simulink model "ofdm"  (R2017b)
settings: Solver=FixedStepDiscrete  StartTime=0.0  StopTime=0.1  RelTol=1e-3
PreLoadFcn:
  | B=18e6;
  | driverChannels = 32;
  | dataChannels = 4096-driverChannels;
  | totalChannels = 4*4096;
  | tau = 100e-9;
  | SNR=30;
  | M=128;
  | Ts = (driverChannels+dataChannels)/B;
InitFcn:
  | B=18e6;
  | driverChannels = 32;
  | dataChannels = 4096-driverChannels;
  | totalChannels = 4096;
  | tau = 100e-9;
  | SNR=15;
  | M=4;
  | Ts = (driverChannels+dataChannels)/B;
undefined symbols (not defined in the file or in its folder): Channels, doppler
libraries: commchan3 x2, dspxfrm3 x2, commdigbbndam3 x2, commrandsrc3 x1, simulink x1, commsink2 x1, dspmathops x1
settings Model: SimulationMode=accelerator  Creator=nschrader  LastModifiedBy=nick
settings SolverCC: AutoInsertRateTranBlk=on
settings DataIOCC: LimitDataPoints=on  SaveOutput=off  SignalLogging=off  SaveTime=off
settings OptimizationCC: LifeSpan=inf
settings DebuggingCC: AlgebraicLoopMsg=error  SingleTaskRateTransMsg=error  AllowSymbolicDim=off  SFUnexpectedBacktrackingDiag=warning  SFNoUnconditionalDefaultTransitionDiag=warning  SFExecutionAtInitializationDiag=none
settings HardwareCC: ProdBitPerLong=64  ProdHWDeviceType=Intel->x86-64 (Linux 64)
settings CodeAppCC: StateflowObjectComments=on
settings GRTTargetCC: TargetLangStandard=C89/C90 (ANSI)  GeneratePreprocessorConditionals=Disable all

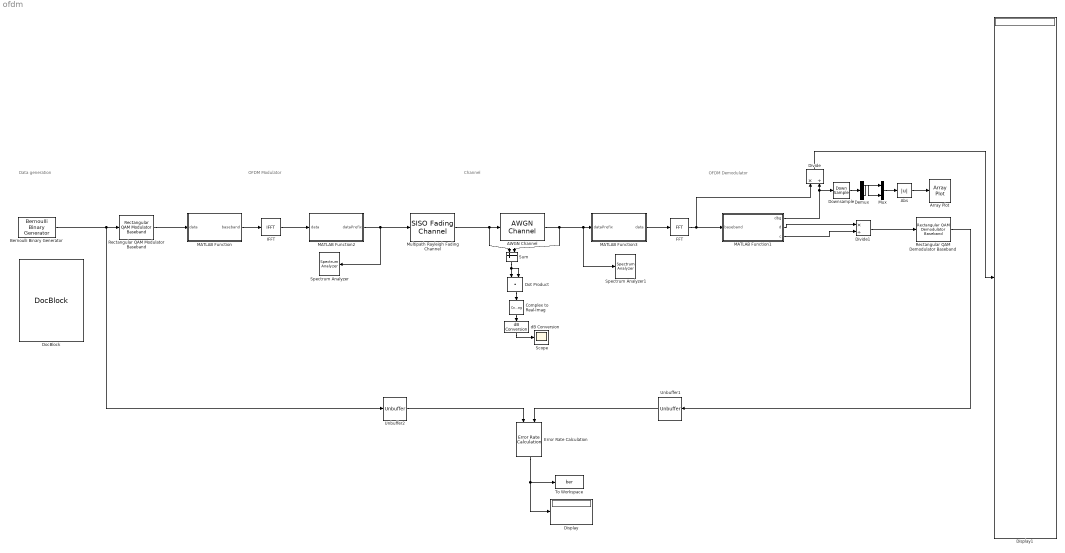
== system ofdm ==
  note: Data generation
  note: OFDM Modulator
  note: Channel
  note: OFDM Demodulator
  AWGN Channel : commchan3/AWGN Channel  InputProcessing=Columns as channels (frame based)  seed=67  noiseMode="Signal to noise ratio  (SNR)"  EbNodB=10  EsNodB=10  SNRdB=SNR  bitsPerSym=1  Ps=(driverChannels+dataChannels)/((totalChannels)^2)  Tsym=1  variance=1
  Abs : Abs
  Array Plot : ArrayPlot
  Bernoulli Binary Generator : commrandsrc3/Bernoulli Binary Generator  ProbabilityOfZero=0.5  SeedSource=Auto  Seed=0  SampleTime=Ts/dataChannels/log2(M)  SamplesPerFrame=dataChannels*log2(M)  OutputDataType=double  SimulateUsing=Code generation
  Complex to Real-Imag : ComplexToRealImag  Output=Real
  Demux : Demux  Outputs=2
  Display : Display
  Display1 : Display
  Divide : Product  Inputs=*/
  Divide1 : Product  Inputs=*/
  DocBlock : simulink/Model-Wide Utilities/DocBlock  DocumentType=Text  mask(DocBlock){}
      content=|
      | Type your documentation here
      mask Display:
      | B = evalin('base', 'B');
      | fprintf(['B = ',num2str(B*1e-6),' MHz\n\n\n\n\n\n\n\n\n\n\n\n\n\n\n\n']);
      | 
      | dataChannels = evalin('base', 'dataChannels');
      | fprintf(['dataChannels = ',num2str(dataChannels), '\n\n\n\n\n\n\n\n\n\n\n\n\n\n']);
      | 
      | totalChannels = evalin('base', 'totalChannels');
      | fprintf(['totalChannels = ',num2str(totalChannels), '\n\n\n\n\n\n\n\n\n\n\n\n']);
      | 
      | driverChannels = evalin('base', 'driverChannels');
      | fprintf(['driverChannels = ',num2str(driverChannels), '\n\n\n\n\n\n\n\n\n\n']);
      | 
      | SNR = evalin('base', 'SNR');
      | fprintf(['SNR = ',num2str(SNR), '\n\n\n\n\n\n\n\n']);
      | 
      | M = evalin('base', 'M');
      | fprintf(['M = ',num2str(M), '\n\n\n\n\n\n']);
      | 
      | Ts = evalin('base', 'Ts');
      | fprintf(['=> Ts = ',num2str(Ts*1e6), ' µs\n\n\n\n']);
      | 
      | rate = log2(M)*dataChannels/Ts/1e6;
      | fprintf(['=> dataRate = ',num2str(rate), ' Mbit/s\n\n']);
      | 
      | capacity = 20*log2(1+10^(SNR/10));
      | fprintf(['=> Efficientcy = ',num2str(100*rate/capacity), ' %%']);
  Dot Product : DotProduct  InputSameDT=on  OutDataTypeStr=Inherit: Inherit via internal rule
  Downsample : DownSample  N=32
  Error Rate Calculation : commsink2/Error Rate Calculation  N=0  st_delay=0  cp_mode=Entire frame  subframe=[]  PMode=Port  WsName=ErrorVec  RsMode2=off  stop=off  numErr=100  maxBits=1e6
  FFT : dspxfrm3/FFT  FFTImplementation=Auto  CompMethod=Table lookup  TableOpt=NEW  TableOptActive=Speed  BitRevOrder=off  Normalize=off  InheritFFTLength=on  FFTLength=Channels  WrapInput=off  roundingMode=Floor  overflowMode=off  firstCoeffDataTypeStr=Inherit: Same word length as input  firstCoeffLastDataTypeStr=Inherit: Same word length as input  outputMin=[]  outputMax=[]
  IFFT : dspxfrm3/IFFT  FFTImplementation=Auto  CompMethod=Table lookup  TableOpt=NEW  TableOptActive=Speed  BitRevOrder=off  cs_in=off  Normalize=on  InheritFFTLength=on  FFTLength=Channels*4  WrapInput=on  mode=Complex  outSamplingMode=Sample based  roundingMode=Floor  overflowMode=off  firstCoeffDataTypeStr=Inherit: Same word length as input  firstCoeffLastDataTypeStr=Inherit: Same word length as input  outputMin=[]  outputMax=[]
      settings: SourceProductName=DSP System Toolbox
  MATLAB Function : MATLAB Function  TreatAsAtomicUnit=on
  MATLAB Function1 : MATLAB Function  TreatAsAtomicUnit=on
  MATLAB Function2 : MATLAB Function  TreatAsAtomicUnit=on
  MATLAB Function3 : MATLAB Function  TreatAsAtomicUnit=on
  Multipath Rayleigh Fading Channel : commchan3/SISO Fading Channel  PathDelays=[0 0.5e-7 1e-7]  AveragePathGains=[0 -3 -6]  NormalizePathGains=on  FadingDistribution=Rayleigh  KFactor=3  DirectPathDopplerShift=0  DirectPathInitialPhase=0  MaximumDopplerShift=40  DopplerSpectrum=doppler('Jakes')  RandomStream=mt19937ar with seed  RandomNumGenerator=shr3cong  Seed=73  PathGainsOutputPort=off  ChannelFilterDelayOutputPort=off  SimulateUsing=Interpreted execution  Visualization=Off  PathsForDopplerDisplay=1  SamplesToDisplay=25%
      settings: SourceProductName=Communications System Toolbox
  Mux : Mux  Inputs=2
  Rectangular QAM Demodulator Baseband : commdigbbndam3/Rectangular QAM Demodulator Baseband  M=M  OutType=Bit  DecType=Hard decision  VarSource=Dialog  Variance=1  Dec=Gray  Mapping=[0:15]  PowType=Average Power  MinDist=2  AvgPow=1  PeakPow=1  Ph=0  outDtype1=Inherit via internal rule  outDtype2=Inherit via internal rule  derotateFactorWordLen=16  derotateFactorDataTypeStr=Inherit: Same word length as input  derotateFactorLastDataTypeStr=Inherit: Same word length as input  denormFactorWordLen=16  denormFactorDataTypeStr=Inherit: Same word length as input  denormFactorLastDataTypeStr=Inherit: Same word length as input  prodOutWordLen=32  prodOutOverflowMode=Wrap  prodOutRoundingMode=Floor  prodOutOvFlMode=off  prodOutOvFlModeLastStrValue=off  sumWordLen=32
  Rectangular QAM Modulator Baseband : commdigbbndam3/Rectangular QAM Modulator Baseband  M=M  InType=Bit  Enc=Gray  Mapping=[0:15]  PowType=Average Power  MinDist=2  AvgPow=1  PeakPow=1  Ph=0  outDtype=double  outWordLen=16  outUDDataType=sfix(16)  outFracLenMode=Best precision  outFracLen=15  outDataTypeStr=double  outLastDataTypeStr=double
  Scope : Scope
  Spectrum Analyzer : SpectrumAnalyzer
  Spectrum Analyzer1 : SpectrumAnalyzer
  Sum : Sum  Inputs=+-
  To Workspace : ToWorkspace  VariableName=ber  SaveFormat=Timeseries  SampleTime=-1
  Unbuffer1 : Unbuffer
  Unbuffer2 : Unbuffer
  dB Conversion : dspmathops/dB Conversion  dBtype=dB  intype=Power  R=1  fuzz=off
      settings: SourceProductName=DSP System Toolbox
  wires:
  Bernoulli Binary Generator/1 -> Rectangular QAM Modulator Baseband/1, Unbuffer2/1
  FFT/1 -> MATLAB Function1/1(baseband), Divide/1
  Error Rate Calculation/1 -> To Workspace/1, Display/1
  Rectangular QAM Demodulator Baseband/1 -> Unbuffer1/1
  Unbuffer2/1 -> Error Rate Calculation/1
  MATLAB Function/1(baseband) -> IFFT/1
  Divide1/1 -> Rectangular QAM Demodulator Baseband/1
  Unbuffer1/1 -> Error Rate Calculation/2
  IFFT/1 -> MATLAB Function2/1(data)
  Multipath Rayleigh Fading Channel/1 -> Sum/1, AWGN Channel/1
  Divide/1 -> Display1/1
  MATLAB Function1/2(d) -> Divide1/1
  MATLAB Function1/3(c) -> Divide1/2
  MATLAB Function1/1(dbg) -> Downsample/1, Divide/2
  MATLAB Function2/1(dataPrefix) -> Multipath Rayleigh Fading Channel/1, Spectrum Analyzer/1
  MATLAB Function3/1(data) -> FFT/1
  AWGN Channel/1 -> Sum/2, Spectrum Analyzer1/1, MATLAB Function3/1(dataPrefix)
  Rectangular QAM Modulator Baseband/1 -> MATLAB Function/1(data)
  Sum/1 -> Dot Product/1, Dot Product/2
  Dot Product/1 -> Complex to Real-Imag/1
  dB Conversion/1 -> Scope/1
  Complex to Real-Imag/1 -> dB Conversion/1
  Downsample/1 -> Demux/1
  Demux/1 -> Mux/2
  Demux/2 -> Mux/1
  Mux/1 -> Abs/1
  Abs/1 -> Array Plot/1

== matlab function ofdm/MATLAB Function1 ==
  data: dbg output size=[totalChannels 1]; baseband input; totalChannels parameter; d output size=[dataChannels 1]; dataChannels parameter; driverChannels parameter; c output size=[dataChannels 1]
function [dbg, d, c] = decompileChannels(baseband, totalChannels, dataChannels, driverChannels)
 % Row vector for using vector concentration
 baseband = baseband';
 
 % Useful variables
 usedChannels = dataChannels + driverChannels;
 deltaChannel = dataChannels/driverChannels;
 
 % Fix variables for indices 
 fDeltaChannel = fix(deltaChannel);
 fUsedChannels_2 = fix(usedChannels/2);
 fDriverChannels_2 = fix(driverChannels/2);
 
 % Helper function
 cones = @(n) complex(ones(1, n));
 czeros = @(n) complex(zeros(1, n));
 nans = @(n) nan(1, n);
 
 % Remove null channels
 driver = czeros(usedChannels);
 driver(1:fUsedChannels_2) = baseband(1:fUsedChannels_2);
 driver(fUsedChannels_2+1:end) = baseband(totalChannels-fUsedChannels_2+1:end);
 
 %Extract data channels
 for j=1:fDriverChannels_2
     for i=(fDeltaChannel+1)*j-1:-1:1
        % Flip vector elements
        driver([i i+1]) = driver([i+1 i]);
        driver([usedChannels-i+1 usedChannels-i]) = driver([usedChannels-i usedChannels-i+1]);
     end
 end
 data = czeros(dataChannels);
 data(1:dataChannels) = driver(fDriverChannels_2+1:fDriverChannels_2+dataChannels);
 
 %Interpolate driver channels
 driver(fDriverChannels_2+1:fDriverChannels_2+dataChannels) = nans(dataChannels);
 for j=fDriverChannels_2:-1:1
     for i=1:(fDeltaChannel+1)*j-1
         % Flip vector elements
        driver([i i+1]) = driver([i+1 i]);
        driver([usedChannels-i+1 usedChannels-i]) = driver([usedChannels-i usedChannels-i+1]);
     end
 end
 coder.extrinsic('fillmissing');
 driver = fillmissing(driver, 'pchip');
 
 %Debug port containing complete channel estimation
 debug = czeros(totalChannels);
 debug(1:fUsedChannels_2) = driver(1:fUsedChannels_2);
 debug(totalChannels-fUsedChannels_2+1:end) = driver(fUsedChannels_2+1:end);
  
 %Extraction of interpolated estimation
 for j=1:fDriverChannels_2
     for i=(fDeltaChannel+1)*j-1:-1:1
        % Flip vector elements
        driver([i i+1]) = driver([i+1 i]);
        driver([usedChannels-i+1 usedChannels-i]) = driver([usedChannels-i usedChannels-i+1]);
     end
 end
 drvs = czeros(dataChannels);
 drvs(1:dataChannels) = driver(fDriverChannels_2+1:fDriverChannels_2+dataChannels);
  
 % Column vector for simulink
 d = data';
 c = drvs';
 dbg = debug';
end

== matlab function ofdm/MATLAB Function ==
  data: data input; baseband output size=[totalChannels 1]; totalChannels parameter; dataChannels parameter; driverChannels parameter
function baseband = compileChannels(data, totalChannels, dataChannels, driverChannels)
 % Row vector for using vector concentration
 data = data';

 % Useful variables
 usedChannels = dataChannels + driverChannels;
 deltaChannel = dataChannels/driverChannels;
 
 % Fix variables for indices 
 fDeltaChannel = fix(deltaChannel);
 fUsedChannels_2 = fix(usedChannels/2);
 fDriverChannels_2 = fix(driverChannels/2);
 
 % Helper function
 cones = @(n) complex(ones(1, n));
 czeros = @(n) complex(zeros(1, n));
 
 %Add driver channels
 driver = [cones(fDriverChannels_2) data cones(fDriverChannels_2)];
 for j=fDriverChannels_2:-1:1
     for i=1:(fDeltaChannel+1)*j-1
         % Flip vector elements
        driver([i i+1]) = driver([i+1 i]);
        driver([usedChannels-i+1 usedChannels-i]) = driver([usedChannels-i usedChannels-i+1]);
     end
 end
  
 % Add null channels
 bb = czeros(totalChannels);
 bb(1:fUsedChannels_2) = driver(1:fUsedChannels_2);
 bb(totalChannels-fUsedChannels_2+1:end) = driver(fUsedChannels_2+1:end);
 
 % Column vector for simulink
 baseband = bb';
end

== matlab function ofdm/MATLAB Function2 ==
  data: data input size=[totalChannels 1]; dataPrefix output; totalChannels parameter; tau parameter; Ts parameter
function dataPrefix = cylicPrefix(data, totalChannels, tau, Ts)
 % Row vector for using vector concentration
 data = data';
 tauPrefix = tau*1.2;
 
 % Calcul du nombre de points du préfixe cyclique en fonction du retard tau
 nbPoints = (tauPrefix*totalChannels)/Ts;
 nbPoints = ceil(nbPoints);
 
 prefix = data(totalChannels-nbPoints+1:end);
 dataPrefix = [ prefix data ]';
end

== matlab function ofdm/MATLAB Function3 ==
  data: dataPrefix input; data output size=[totalChannels 1]; totalChannels parameter; tau parameter; Ts parameter
function data = cylicPrefix(dataPrefix, totalChannels, tau, Ts)
 % Row vector for using vector concentration
 dataPrefix = dataPrefix';
 tauPrefix = tau*1.2;
 
 % Calcul du nombre de points du préfixe cyclique en fonction du retard tau
 nbPoints = (tauPrefix*totalChannels)/Ts;
 nbPoints = ceil(nbPoints);
 
 data = dataPrefix(nbPoints+1:end)';
end
